simulink model "TST_RmtAPP_ChkSig"  (R2016b)
settings: Solver=FixedStepDiscrete  StartTime=0.0  StopTime=simTime  FixedStep=sampleTime  RelTol=1e-3
values from neighbouring files (symbols this model uses):
  testCase = 1    [initTST_RmtAPP_ChkSig_001.m]    (also in initTST_RmtAPP_ChkSig_002.m = 2; initTST_RmtAPP_ChkSig_003.m = 3; initTST_RmtAPP_ChkSig_004.m = 4; initTST_RmtAPP_ChkSig_005.m = 5)
libraries: simulink x11, UnitTest_Lib x5
settings Model: Creator=bianxuyin  LastModifiedBy=bianxuyin
settings DebuggingCC: SignalRangeChecking=error

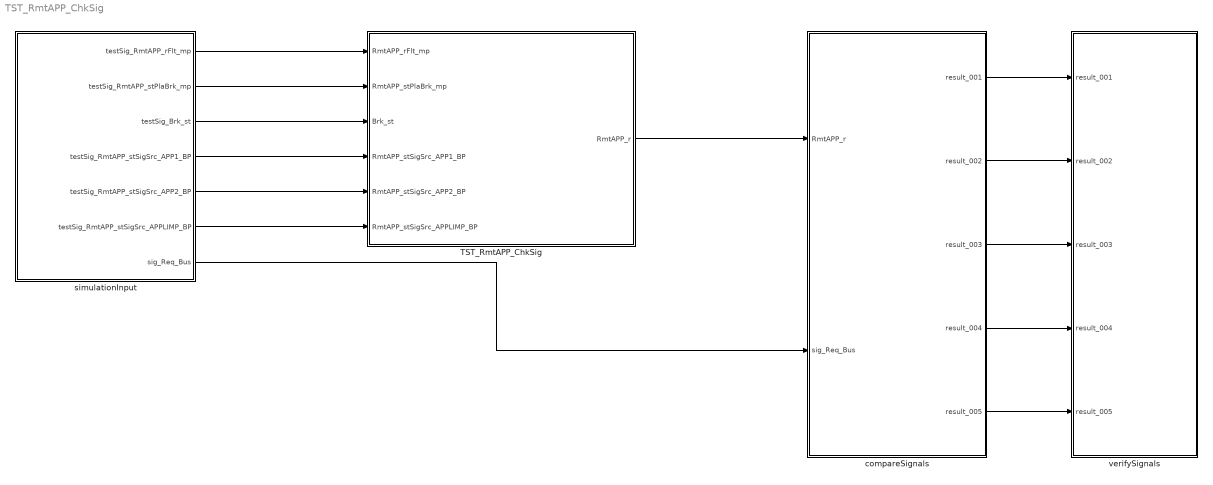
== system TST_RmtAPP_ChkSig ==
  TST_RmtAPP_ChkSig : Subsystem
  compareSignals : Subsystem
  simulationInput : Subsystem
  verifySignals : Subsystem
  wires:
  simulationInput/1(testSig_RmtAPP_rFlt_mp) -> TST_RmtAPP_ChkSig/1(RmtAPP_rFlt_mp)
  simulationInput/2(testSig_RmtAPP_stPlaBrk_mp) -> TST_RmtAPP_ChkSig/2(RmtAPP_stPlaBrk_mp)
  simulationInput/3(testSig_Brk_st) -> TST_RmtAPP_ChkSig/3(Brk_st)
  simulationInput/4(testSig_RmtAPP_stSigSrc_APP1_BP) -> TST_RmtAPP_ChkSig/4(RmtAPP_stSigSrc_APP1_BP)
  simulationInput/5(testSig_RmtAPP_stSigSrc_APP2_BP) -> TST_RmtAPP_ChkSig/5(RmtAPP_stSigSrc_APP2_BP)
  simulationInput/6(testSig_RmtAPP_stSigSrc_APPLIMP_BP) -> TST_RmtAPP_ChkSig/6(RmtAPP_stSigSrc_APPLIMP_BP)
  TST_RmtAPP_ChkSig/1(RmtAPP_r) -> compareSignals/1(RmtAPP_r)
  simulationInput/7(sig_Req_Bus) -> compareSignals/2(sig_Req_Bus)
  compareSignals/1(result_001) -> verifySignals/1(result_001)
  compareSignals/2(result_002) -> verifySignals/2(result_002)
  compareSignals/3(result_003) -> verifySignals/3(result_003)
  compareSignals/4(result_004) -> verifySignals/4(result_004)
  compareSignals/5(result_005) -> verifySignals/5(result_005)

== system TST_RmtAPP_ChkSig/TST_RmtAPP_ChkSig ==
  RmtAPP_rFlt_mp : Inport
  RmtAPP_stPlaBrk_mp : Inport  Port=2
  Brk_st : Inport  Port=3
  RmtAPP_stSigSrc_APP1_BP : Inport  Port=4
  RmtAPP_stSigSrc_APP2_BP : Inport  Port=5
  RmtAPP_stSigSrc_APPLIMP_BP : Inport  Port=6
  Function_Call : simulink/Ports & Subsystems/Function-Call Generator  sample_time=sampleTime  numberOfIterations=1
  RmtAPP_ChkSig : ModelReference  ModelNameDialog=RmtAPP_ChkSig  SimulationMode=Normal  ModelReferenceVersion=1.13  TriggerPortName=function  TriggerPortTriggerType=function-call  TriggerPortStatesWhenEnabling=held
  RmtAPP_r : Outport
  wires:
  Function_Call/1 -> RmtAPP_ChkSig/Trigger
  RmtAPP_rFlt_mp/1 -> RmtAPP_ChkSig/1
  RmtAPP_stPlaBrk_mp/1 -> RmtAPP_ChkSig/2
  Brk_st/1 -> RmtAPP_ChkSig/3
  RmtAPP_stSigSrc_APP1_BP/1 -> RmtAPP_ChkSig/4
  RmtAPP_stSigSrc_APP2_BP/1 -> RmtAPP_ChkSig/5
  RmtAPP_stSigSrc_APPLIMP_BP/1 -> RmtAPP_ChkSig/6
  RmtAPP_ChkSig/1 -> RmtAPP_r/1

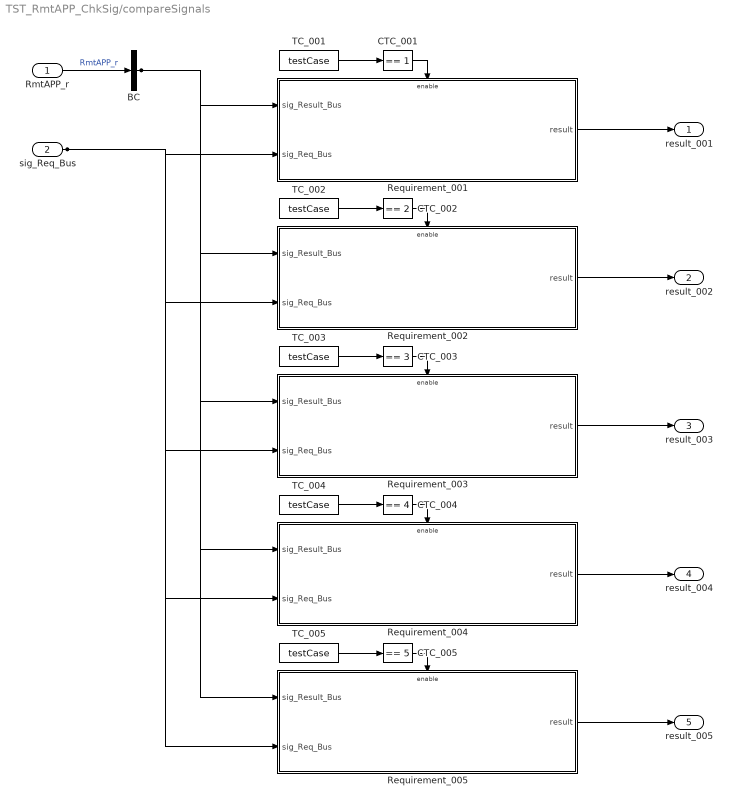
== system TST_RmtAPP_ChkSig/compareSignals ==
  RmtAPP_r : Inport
  sig_Req_Bus : Inport  Port=2
  BC : BusCreator  Inputs=1
  CTC_001 : simulink/Logic and Bit Operations/Compare To Constant  relop===  const=1  OutDataTypeStr=boolean
  CTC_002 : simulink/Logic and Bit Operations/Compare To Constant  relop===  const=2  OutDataTypeStr=boolean
  CTC_003 : simulink/Logic and Bit Operations/Compare To Constant  relop===  const=3  OutDataTypeStr=boolean
  CTC_004 : simulink/Logic and Bit Operations/Compare To Constant  relop===  const=4  OutDataTypeStr=boolean
  CTC_005 : simulink/Logic and Bit Operations/Compare To Constant  relop===  const=5  OutDataTypeStr=boolean
  Requirement_001 : Subsystem
  Requirement_002 : Subsystem
  Requirement_003 : Subsystem
  Requirement_004 : Subsystem
  Requirement_005 : Subsystem
  TC_001 : Constant  Value=testCase
  TC_002 : Constant  Value=testCase
  TC_003 : Constant  Value=testCase
  TC_004 : Constant  Value=testCase
  TC_005 : Constant  Value=testCase
  result_001 : Outport
  result_002 : Outport  Port=2
  result_003 : Outport  Port=3
  result_004 : Outport  Port=4
  result_005 : Outport  Port=5
  wires:
  RmtAPP_r/1 -> BC/1  "RmtAPP_r"
  TC_001/1 -> CTC_001/1
  CTC_001/1 -> Requirement_001/Enable
  sig_Req_Bus/1 -> Requirement_001/2(sig_Req_Bus), Requirement_002/2(sig_Req_Bus), Requirement_003/2(sig_Req_Bus), Requirement_004/2(sig_Req_Bus), Requirement_005/2(sig_Req_Bus)
  BC/1 -> Requirement_001/1(sig_Result_Bus), Requirement_002/1(sig_Result_Bus), Requirement_003/1(sig_Result_Bus), Requirement_004/1(sig_Result_Bus), Requirement_005/1(sig_Result_Bus)
  Requirement_001/1(result) -> result_001/1
  TC_002/1 -> CTC_002/1
  CTC_002/1 -> Requirement_002/Enable
  Requirement_002/1(result) -> result_002/1
  TC_003/1 -> CTC_003/1
  CTC_003/1 -> Requirement_003/Enable
  Requirement_003/1(result) -> result_003/1
  TC_004/1 -> CTC_004/1
  CTC_004/1 -> Requirement_004/Enable
  Requirement_004/1(result) -> result_004/1
  TC_005/1 -> CTC_005/1
  CTC_005/1 -> Requirement_005/Enable
  Requirement_005/1(result) -> result_005/1

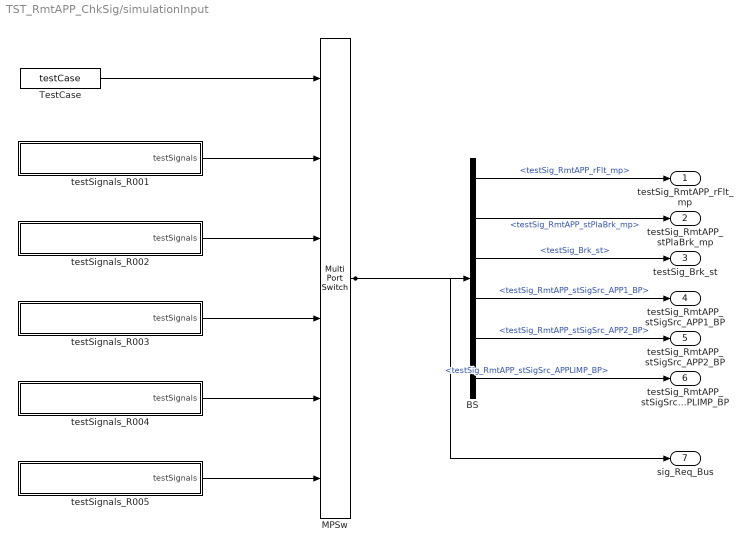
== system TST_RmtAPP_ChkSig/simulationInput ==
  BS : BusSelector  OutputSignals=testSig_RmtAPP_rFlt_mp,testSig_RmtAPP_stPlaBrk_mp,testSig_Brk_st,testSig_RmtAPP_stSigSrc_APP1_BP,testSig_RmtAPP_stSigSrc_APP2_BP,testSig_RmtAPP_stSigSrc_APPLIMP_BP
  MPSw : MultiPortSwitch  Inputs=5  SaturateOnIntegerOverflow=on  InputSameDT=on
  TestCase : Constant  Value=testCase
  testSignals_R001 : Subsystem
  testSignals_R002 : Subsystem
  testSignals_R003 : Subsystem
  testSignals_R004 : Subsystem
  testSignals_R005 : Subsystem
  testSig_RmtAPP_rFlt_mp : Outport
  testSig_RmtAPP_stPlaBrk_mp : Outport  Port=2
  testSig_Brk_st : Outport  Port=3
  testSig_RmtAPP_stSigSrc_APP1_BP : Outport  Port=4
  testSig_RmtAPP_stSigSrc_APP2_BP : Outport  Port=5
  testSig_RmtAPP_stSigSrc_APPLIMP_BP : Outport  Port=6
  sig_Req_Bus : Outport  Port=7
  wires:
  BS/1 -> testSig_RmtAPP_rFlt_mp/1  "<testSig_RmtAPP_rFlt_mp>"
  BS/2 -> testSig_RmtAPP_stPlaBrk_mp/1  "<testSig_RmtAPP_stPlaBrk_mp>"
  BS/3 -> testSig_Brk_st/1  "<testSig_Brk_st>"
  BS/4 -> testSig_RmtAPP_stSigSrc_APP1_BP/1  "<testSig_RmtAPP_stSigSrc_APP1_BP>"
  BS/5 -> testSig_RmtAPP_stSigSrc_APP2_BP/1  "<testSig_RmtAPP_stSigSrc_APP2_BP>"
  BS/6 -> testSig_RmtAPP_stSigSrc_APPLIMP_BP/1  "<testSig_RmtAPP_stSigSrc_APPLIMP_BP>"
  MPSw/1 -> BS/1, sig_Req_Bus/1
  TestCase/1 -> MPSw/1
  testSignals_R001/1(testSignals) -> MPSw/2
  testSignals_R002/1(testSignals) -> MPSw/3
  testSignals_R003/1(testSignals) -> MPSw/4
  testSignals_R004/1(testSignals) -> MPSw/5
  testSignals_R005/1(testSignals) -> MPSw/6

== system TST_RmtAPP_ChkSig/verifySignals ==
  result_001 : Inport
  result_002 : Inport  Port=2
  result_003 : Inport  Port=3
  result_004 : Inport  Port=4
  result_005 : Inport  Port=5
  Assertion_001 : Assertion  Enabled=off
  Assertion_002 : Assertion  Enabled=off
  Assertion_003 : Assertion  Enabled=off
  Assertion_004 : Assertion  Enabled=off
  Assertion_005 : Assertion  Enabled=off
  wires:
  result_001/1 -> Assertion_001/1
  result_002/1 -> Assertion_002/1
  result_003/1 -> Assertion_003/1
  result_004/1 -> Assertion_004/1
  result_005/1 -> Assertion_005/1

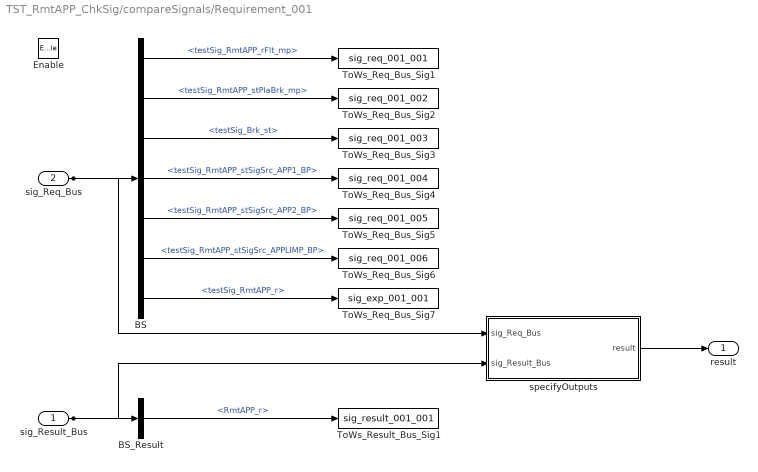
== system TST_RmtAPP_ChkSig/compareSignals/Requirement_001 ==
  sig_Result_Bus : Inport
  sig_Req_Bus : Inport  Port=2
  Enable : EnablePort
  BS : BusSelector  OutputSignals=testSig_RmtAPP_rFlt_mp,testSig_RmtAPP_stPlaBrk_mp,testSig_Brk_st,testSig_RmtAPP_stSigSrc_APP1_BP,testSig_RmtAPP_stSigSrc_APP2_BP,testSig_RmtAPP_stSigSrc_APPLIMP_BP,testSig_RmtAPP_r
  BS_Result : BusSelector  OutputSignals=RmtAPP_r
  ToWs_Req_Bus_Sig1 : ToWorkspace  VariableName=sig_req_001_001  SaveFormat=Structure With Time
  ToWs_Req_Bus_Sig2 : ToWorkspace  VariableName=sig_req_001_002  SaveFormat=Structure With Time
  ToWs_Req_Bus_Sig3 : ToWorkspace  VariableName=sig_req_001_003  SaveFormat=Structure With Time
  ToWs_Req_Bus_Sig4 : ToWorkspace  VariableName=sig_req_001_004  SaveFormat=Structure With Time
  ToWs_Req_Bus_Sig5 : ToWorkspace  VariableName=sig_req_001_005  SaveFormat=Structure With Time
  ToWs_Req_Bus_Sig6 : ToWorkspace  VariableName=sig_req_001_006  SaveFormat=Structure With Time
  ToWs_Req_Bus_Sig7 : ToWorkspace  VariableName=sig_exp_001_001  SaveFormat=Structure With Time
  ToWs_Result_Bus_Sig1 : ToWorkspace  VariableName=sig_result_001_001  SaveFormat=Structure With Time
  specifyOutputs : Subsystem
  result : Outport
  wires:
  sig_Req_Bus/1 -> BS/1, specifyOutputs/1(sig_Req_Bus)
  BS/1 -> ToWs_Req_Bus_Sig1/1  "<testSig_RmtAPP_rFlt_mp>"
  BS/2 -> ToWs_Req_Bus_Sig2/1  "<testSig_RmtAPP_stPlaBrk_mp>"
  BS/3 -> ToWs_Req_Bus_Sig3/1  "<testSig_Brk_st>"
  BS/4 -> ToWs_Req_Bus_Sig4/1  "<testSig_RmtAPP_stSigSrc_APP1_BP>"
  BS/5 -> ToWs_Req_Bus_Sig5/1  "<testSig_RmtAPP_stSigSrc_APP2_BP>"
  BS/6 -> ToWs_Req_Bus_Sig6/1  "<testSig_RmtAPP_stSigSrc_APPLIMP_BP>"
  BS/7 -> ToWs_Req_Bus_Sig7/1  "<testSig_RmtAPP_r>"
  sig_Result_Bus/1 -> BS_Result/1, specifyOutputs/2(sig_Result_Bus)
  BS_Result/1 -> ToWs_Result_Bus_Sig1/1  "<RmtAPP_r>"
  specifyOutputs/1(result) -> result/1

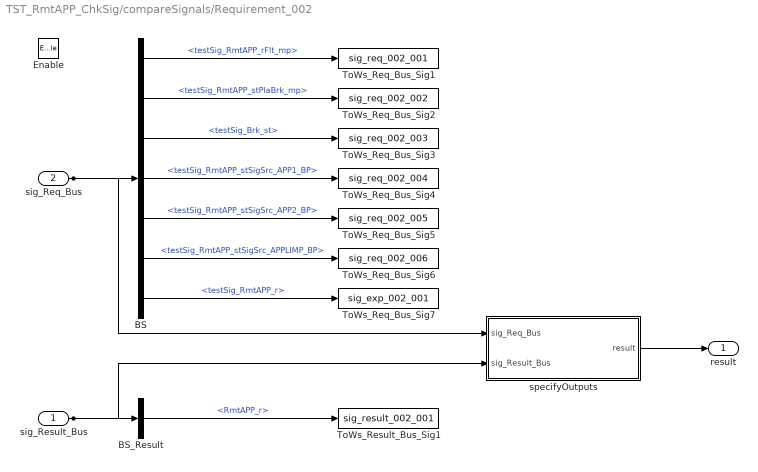
== system TST_RmtAPP_ChkSig/compareSignals/Requirement_002 ==
  sig_Result_Bus : Inport
  sig_Req_Bus : Inport  Port=2
  Enable : EnablePort
  BS : BusSelector  OutputSignals=testSig_RmtAPP_rFlt_mp,testSig_RmtAPP_stPlaBrk_mp,testSig_Brk_st,testSig_RmtAPP_stSigSrc_APP1_BP,testSig_RmtAPP_stSigSrc_APP2_BP,testSig_RmtAPP_stSigSrc_APPLIMP_BP,testSig_RmtAPP_r
  BS_Result : BusSelector  OutputSignals=RmtAPP_r
  ToWs_Req_Bus_Sig1 : ToWorkspace  VariableName=sig_req_002_001  SaveFormat=Structure With Time
  ToWs_Req_Bus_Sig2 : ToWorkspace  VariableName=sig_req_002_002  SaveFormat=Structure With Time
  ToWs_Req_Bus_Sig3 : ToWorkspace  VariableName=sig_req_002_003  SaveFormat=Structure With Time
  ToWs_Req_Bus_Sig4 : ToWorkspace  VariableName=sig_req_002_004  SaveFormat=Structure With Time
  ToWs_Req_Bus_Sig5 : ToWorkspace  VariableName=sig_req_002_005  SaveFormat=Structure With Time
  ToWs_Req_Bus_Sig6 : ToWorkspace  VariableName=sig_req_002_006  SaveFormat=Structure With Time
  ToWs_Req_Bus_Sig7 : ToWorkspace  VariableName=sig_exp_002_001  SaveFormat=Structure With Time
  ToWs_Result_Bus_Sig1 : ToWorkspace  VariableName=sig_result_002_001  SaveFormat=Structure With Time
  specifyOutputs : Subsystem
  result : Outport
  wires:
  sig_Req_Bus/1 -> BS/1, specifyOutputs/1(sig_Req_Bus)
  BS/1 -> ToWs_Req_Bus_Sig1/1  "<testSig_RmtAPP_rFlt_mp>"
  BS/2 -> ToWs_Req_Bus_Sig2/1  "<testSig_RmtAPP_stPlaBrk_mp>"
  BS/3 -> ToWs_Req_Bus_Sig3/1  "<testSig_Brk_st>"
  BS/4 -> ToWs_Req_Bus_Sig4/1  "<testSig_RmtAPP_stSigSrc_APP1_BP>"
  BS/5 -> ToWs_Req_Bus_Sig5/1  "<testSig_RmtAPP_stSigSrc_APP2_BP>"
  BS/6 -> ToWs_Req_Bus_Sig6/1  "<testSig_RmtAPP_stSigSrc_APPLIMP_BP>"
  BS/7 -> ToWs_Req_Bus_Sig7/1  "<testSig_RmtAPP_r>"
  sig_Result_Bus/1 -> BS_Result/1, specifyOutputs/2(sig_Result_Bus)
  BS_Result/1 -> ToWs_Result_Bus_Sig1/1  "<RmtAPP_r>"
  specifyOutputs/1(result) -> result/1

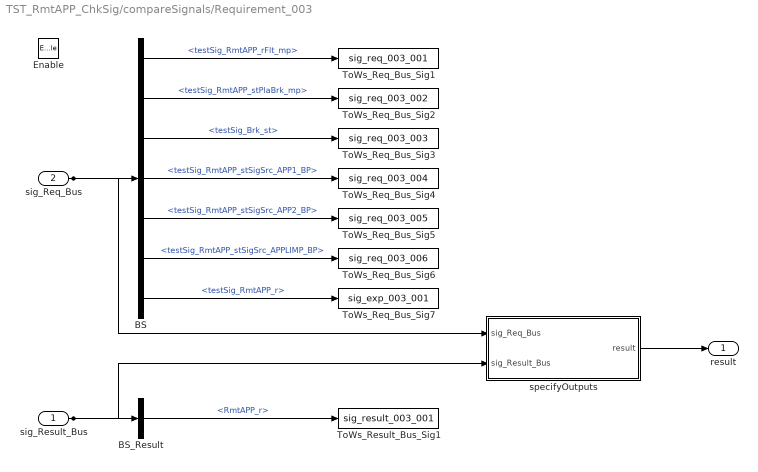
== system TST_RmtAPP_ChkSig/compareSignals/Requirement_003 ==
  sig_Result_Bus : Inport
  sig_Req_Bus : Inport  Port=2
  Enable : EnablePort
  BS : BusSelector  OutputSignals=testSig_RmtAPP_rFlt_mp,testSig_RmtAPP_stPlaBrk_mp,testSig_Brk_st,testSig_RmtAPP_stSigSrc_APP1_BP,testSig_RmtAPP_stSigSrc_APP2_BP,testSig_RmtAPP_stSigSrc_APPLIMP_BP,testSig_RmtAPP_r
  BS_Result : BusSelector  OutputSignals=RmtAPP_r
  ToWs_Req_Bus_Sig1 : ToWorkspace  VariableName=sig_req_003_001  SaveFormat=Structure With Time
  ToWs_Req_Bus_Sig2 : ToWorkspace  VariableName=sig_req_003_002  SaveFormat=Structure With Time
  ToWs_Req_Bus_Sig3 : ToWorkspace  VariableName=sig_req_003_003  SaveFormat=Structure With Time
  ToWs_Req_Bus_Sig4 : ToWorkspace  VariableName=sig_req_003_004  SaveFormat=Structure With Time
  ToWs_Req_Bus_Sig5 : ToWorkspace  VariableName=sig_req_003_005  SaveFormat=Structure With Time
  ToWs_Req_Bus_Sig6 : ToWorkspace  VariableName=sig_req_003_006  SaveFormat=Structure With Time
  ToWs_Req_Bus_Sig7 : ToWorkspace  VariableName=sig_exp_003_001  SaveFormat=Structure With Time
  ToWs_Result_Bus_Sig1 : ToWorkspace  VariableName=sig_result_003_001  SaveFormat=Structure With Time
  specifyOutputs : Subsystem
  result : Outport
  wires:
  sig_Req_Bus/1 -> BS/1, specifyOutputs/1(sig_Req_Bus)
  BS/1 -> ToWs_Req_Bus_Sig1/1  "<testSig_RmtAPP_rFlt_mp>"
  BS/2 -> ToWs_Req_Bus_Sig2/1  "<testSig_RmtAPP_stPlaBrk_mp>"
  BS/3 -> ToWs_Req_Bus_Sig3/1  "<testSig_Brk_st>"
  BS/4 -> ToWs_Req_Bus_Sig4/1  "<testSig_RmtAPP_stSigSrc_APP1_BP>"
  BS/5 -> ToWs_Req_Bus_Sig5/1  "<testSig_RmtAPP_stSigSrc_APP2_BP>"
  BS/6 -> ToWs_Req_Bus_Sig6/1  "<testSig_RmtAPP_stSigSrc_APPLIMP_BP>"
  BS/7 -> ToWs_Req_Bus_Sig7/1  "<testSig_RmtAPP_r>"
  sig_Result_Bus/1 -> BS_Result/1, specifyOutputs/2(sig_Result_Bus)
  BS_Result/1 -> ToWs_Result_Bus_Sig1/1  "<RmtAPP_r>"
  specifyOutputs/1(result) -> result/1

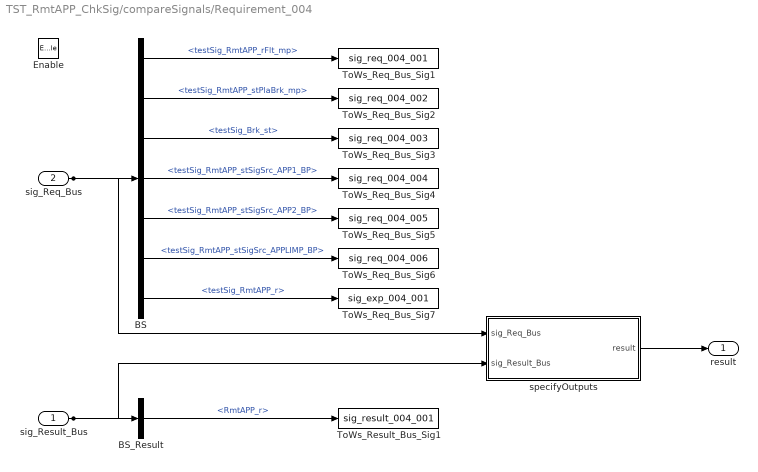
== system TST_RmtAPP_ChkSig/compareSignals/Requirement_004 ==
  sig_Result_Bus : Inport
  sig_Req_Bus : Inport  Port=2
  Enable : EnablePort
  BS : BusSelector  OutputSignals=testSig_RmtAPP_rFlt_mp,testSig_RmtAPP_stPlaBrk_mp,testSig_Brk_st,testSig_RmtAPP_stSigSrc_APP1_BP,testSig_RmtAPP_stSigSrc_APP2_BP,testSig_RmtAPP_stSigSrc_APPLIMP_BP,testSig_RmtAPP_r
  BS_Result : BusSelector  OutputSignals=RmtAPP_r
  ToWs_Req_Bus_Sig1 : ToWorkspace  VariableName=sig_req_004_001  SaveFormat=Structure With Time
  ToWs_Req_Bus_Sig2 : ToWorkspace  VariableName=sig_req_004_002  SaveFormat=Structure With Time
  ToWs_Req_Bus_Sig3 : ToWorkspace  VariableName=sig_req_004_003  SaveFormat=Structure With Time
  ToWs_Req_Bus_Sig4 : ToWorkspace  VariableName=sig_req_004_004  SaveFormat=Structure With Time
  ToWs_Req_Bus_Sig5 : ToWorkspace  VariableName=sig_req_004_005  SaveFormat=Structure With Time
  ToWs_Req_Bus_Sig6 : ToWorkspace  VariableName=sig_req_004_006  SaveFormat=Structure With Time
  ToWs_Req_Bus_Sig7 : ToWorkspace  VariableName=sig_exp_004_001  SaveFormat=Structure With Time
  ToWs_Result_Bus_Sig1 : ToWorkspace  VariableName=sig_result_004_001  SaveFormat=Structure With Time
  specifyOutputs : Subsystem
  result : Outport
  wires:
  sig_Req_Bus/1 -> BS/1, specifyOutputs/1(sig_Req_Bus)
  BS/1 -> ToWs_Req_Bus_Sig1/1  "<testSig_RmtAPP_rFlt_mp>"
  BS/2 -> ToWs_Req_Bus_Sig2/1  "<testSig_RmtAPP_stPlaBrk_mp>"
  BS/3 -> ToWs_Req_Bus_Sig3/1  "<testSig_Brk_st>"
  BS/4 -> ToWs_Req_Bus_Sig4/1  "<testSig_RmtAPP_stSigSrc_APP1_BP>"
  BS/5 -> ToWs_Req_Bus_Sig5/1  "<testSig_RmtAPP_stSigSrc_APP2_BP>"
  BS/6 -> ToWs_Req_Bus_Sig6/1  "<testSig_RmtAPP_stSigSrc_APPLIMP_BP>"
  BS/7 -> ToWs_Req_Bus_Sig7/1  "<testSig_RmtAPP_r>"
  sig_Result_Bus/1 -> BS_Result/1, specifyOutputs/2(sig_Result_Bus)
  BS_Result/1 -> ToWs_Result_Bus_Sig1/1  "<RmtAPP_r>"
  specifyOutputs/1(result) -> result/1

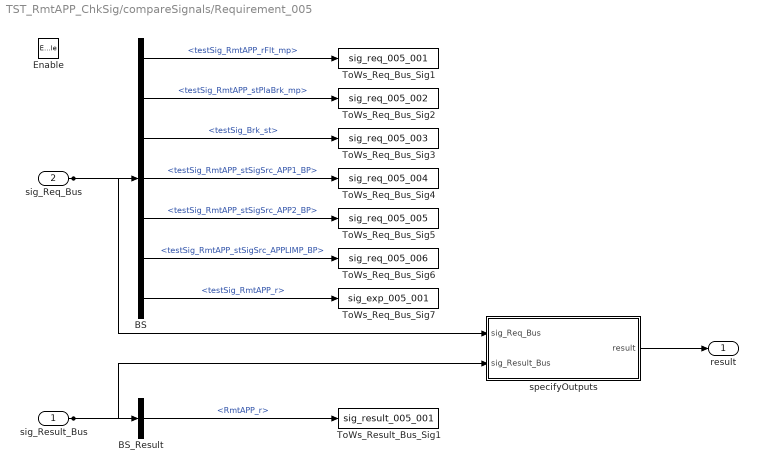
== system TST_RmtAPP_ChkSig/compareSignals/Requirement_005 ==
  sig_Result_Bus : Inport
  sig_Req_Bus : Inport  Port=2
  Enable : EnablePort
  BS : BusSelector  OutputSignals=testSig_RmtAPP_rFlt_mp,testSig_RmtAPP_stPlaBrk_mp,testSig_Brk_st,testSig_RmtAPP_stSigSrc_APP1_BP,testSig_RmtAPP_stSigSrc_APP2_BP,testSig_RmtAPP_stSigSrc_APPLIMP_BP,testSig_RmtAPP_r
  BS_Result : BusSelector  OutputSignals=RmtAPP_r
  ToWs_Req_Bus_Sig1 : ToWorkspace  VariableName=sig_req_005_001  SaveFormat=Structure With Time
  ToWs_Req_Bus_Sig2 : ToWorkspace  VariableName=sig_req_005_002  SaveFormat=Structure With Time
  ToWs_Req_Bus_Sig3 : ToWorkspace  VariableName=sig_req_005_003  SaveFormat=Structure With Time
  ToWs_Req_Bus_Sig4 : ToWorkspace  VariableName=sig_req_005_004  SaveFormat=Structure With Time
  ToWs_Req_Bus_Sig5 : ToWorkspace  VariableName=sig_req_005_005  SaveFormat=Structure With Time
  ToWs_Req_Bus_Sig6 : ToWorkspace  VariableName=sig_req_005_006  SaveFormat=Structure With Time
  ToWs_Req_Bus_Sig7 : ToWorkspace  VariableName=sig_exp_005_001  SaveFormat=Structure With Time
  ToWs_Result_Bus_Sig1 : ToWorkspace  VariableName=sig_result_005_001  SaveFormat=Structure With Time
  specifyOutputs : Subsystem
  result : Outport
  wires:
  sig_Req_Bus/1 -> BS/1, specifyOutputs/1(sig_Req_Bus)
  BS/1 -> ToWs_Req_Bus_Sig1/1  "<testSig_RmtAPP_rFlt_mp>"
  BS/2 -> ToWs_Req_Bus_Sig2/1  "<testSig_RmtAPP_stPlaBrk_mp>"
  BS/3 -> ToWs_Req_Bus_Sig3/1  "<testSig_Brk_st>"
  BS/4 -> ToWs_Req_Bus_Sig4/1  "<testSig_RmtAPP_stSigSrc_APP1_BP>"
  BS/5 -> ToWs_Req_Bus_Sig5/1  "<testSig_RmtAPP_stSigSrc_APP2_BP>"
  BS/6 -> ToWs_Req_Bus_Sig6/1  "<testSig_RmtAPP_stSigSrc_APPLIMP_BP>"
  BS/7 -> ToWs_Req_Bus_Sig7/1  "<testSig_RmtAPP_r>"
  sig_Result_Bus/1 -> BS_Result/1, specifyOutputs/2(sig_Result_Bus)
  BS_Result/1 -> ToWs_Result_Bus_Sig1/1  "<RmtAPP_r>"
  specifyOutputs/1(result) -> result/1

== system TST_RmtAPP_ChkSig/simulationInput/testSignals_R001 ==
  BC : BusCreator  Inputs=7
  spec_Brk_st : FromWorkspace  VariableName=testSig_Brk_st  Interpolate=off  OutputAfterFinalValue=Holding final value
  spec_RmtAPP_r : FromWorkspace  VariableName=testSig_RmtAPP_r  Interpolate=off  OutputAfterFinalValue=Holding final value
  spec_RmtAPP_rFlt_mp : FromWorkspace  VariableName=testSig_RmtAPP_rFlt_mp  Interpolate=off  OutputAfterFinalValue=Holding final value
  spec_RmtAPP_stPlaBrk_mp : FromWorkspace  VariableName=testSig_RmtAPP_stPlaBrk_mp  Interpolate=off  OutputAfterFinalValue=Holding final value
  spec_RmtAPP_stSigSrc_APP1_BP : FromWorkspace  VariableName=testSig_RmtAPP_stSigSrc_APP1_BP  Interpolate=off  OutputAfterFinalValue=Holding final value
  spec_RmtAPP_stSigSrc_APP2_BP : FromWorkspace  VariableName=testSig_RmtAPP_stSigSrc_APP2_BP  Interpolate=off  OutputAfterFinalValue=Holding final value
  spec_RmtAPP_stSigSrc_APPLIMP_BP : FromWorkspace  VariableName=testSig_RmtAPP_stSigSrc_APPLIMP_BP  Interpolate=off  OutputAfterFinalValue=Holding final value
  testSignals : Outport
  wires:
  BC/1 -> testSignals/1
  spec_RmtAPP_rFlt_mp/1 -> BC/1  "testSig_RmtAPP_rFlt_mp"
  spec_RmtAPP_stPlaBrk_mp/1 -> BC/2  "testSig_RmtAPP_stPlaBrk_mp"
  spec_Brk_st/1 -> BC/3  "testSig_Brk_st"
  spec_RmtAPP_stSigSrc_APP1_BP/1 -> BC/4  "testSig_RmtAPP_stSigSrc_APP1_BP"
  spec_RmtAPP_stSigSrc_APP2_BP/1 -> BC/5  "testSig_RmtAPP_stSigSrc_APP2_BP"
  spec_RmtAPP_stSigSrc_APPLIMP_BP/1 -> BC/6  "testSig_RmtAPP_stSigSrc_APPLIMP_BP"
  spec_RmtAPP_r/1 -> BC/7  "testSig_RmtAPP_r"

== system TST_RmtAPP_ChkSig/simulationInput/testSignals_R002 ==
  BC : BusCreator  Inputs=7
  spec_Brk_st : FromWorkspace  VariableName=testSig_Brk_st  Interpolate=off  OutputAfterFinalValue=Holding final value
  spec_RmtAPP_r : FromWorkspace  VariableName=testSig_RmtAPP_r  Interpolate=off  OutputAfterFinalValue=Holding final value
  spec_RmtAPP_rFlt_mp : FromWorkspace  VariableName=testSig_RmtAPP_rFlt_mp  Interpolate=off  OutputAfterFinalValue=Holding final value
  spec_RmtAPP_stPlaBrk_mp : FromWorkspace  VariableName=testSig_RmtAPP_stPlaBrk_mp  Interpolate=off  OutputAfterFinalValue=Holding final value
  spec_RmtAPP_stSigSrc_APP1_BP : FromWorkspace  VariableName=testSig_RmtAPP_stSigSrc_APP1_BP  Interpolate=off  OutputAfterFinalValue=Holding final value
  spec_RmtAPP_stSigSrc_APP2_BP : FromWorkspace  VariableName=testSig_RmtAPP_stSigSrc_APP2_BP  Interpolate=off  OutputAfterFinalValue=Holding final value
  spec_RmtAPP_stSigSrc_APPLIMP_BP : FromWorkspace  VariableName=testSig_RmtAPP_stSigSrc_APPLIMP_BP  Interpolate=off  OutputAfterFinalValue=Holding final value
  testSignals : Outport
  wires:
  BC/1 -> testSignals/1
  spec_RmtAPP_rFlt_mp/1 -> BC/1  "testSig_RmtAPP_rFlt_mp"
  spec_RmtAPP_stPlaBrk_mp/1 -> BC/2  "testSig_RmtAPP_stPlaBrk_mp"
  spec_Brk_st/1 -> BC/3  "testSig_Brk_st"
  spec_RmtAPP_stSigSrc_APP1_BP/1 -> BC/4  "testSig_RmtAPP_stSigSrc_APP1_BP"
  spec_RmtAPP_stSigSrc_APP2_BP/1 -> BC/5  "testSig_RmtAPP_stSigSrc_APP2_BP"
  spec_RmtAPP_stSigSrc_APPLIMP_BP/1 -> BC/6  "testSig_RmtAPP_stSigSrc_APPLIMP_BP"
  spec_RmtAPP_r/1 -> BC/7  "testSig_RmtAPP_r"

== system TST_RmtAPP_ChkSig/simulationInput/testSignals_R003 ==
  BC : BusCreator  Inputs=7
  spec_Brk_st : FromWorkspace  VariableName=testSig_Brk_st  Interpolate=off  OutputAfterFinalValue=Holding final value
  spec_RmtAPP_r : FromWorkspace  VariableName=testSig_RmtAPP_r  Interpolate=off  OutputAfterFinalValue=Holding final value
  spec_RmtAPP_rFlt_mp : FromWorkspace  VariableName=testSig_RmtAPP_rFlt_mp  Interpolate=off  OutputAfterFinalValue=Holding final value
  spec_RmtAPP_stPlaBrk_mp : FromWorkspace  VariableName=testSig_RmtAPP_stPlaBrk_mp  Interpolate=off  OutputAfterFinalValue=Holding final value
  spec_RmtAPP_stSigSrc_APP1_BP : FromWorkspace  VariableName=testSig_RmtAPP_stSigSrc_APP1_BP  Interpolate=off  OutputAfterFinalValue=Holding final value
  spec_RmtAPP_stSigSrc_APP2_BP : FromWorkspace  VariableName=testSig_RmtAPP_stSigSrc_APP2_BP  Interpolate=off  OutputAfterFinalValue=Holding final value
  spec_RmtAPP_stSigSrc_APPLIMP_BP : FromWorkspace  VariableName=testSig_RmtAPP_stSigSrc_APPLIMP_BP  Interpolate=off  OutputAfterFinalValue=Holding final value
  testSignals : Outport
  wires:
  BC/1 -> testSignals/1
  spec_RmtAPP_rFlt_mp/1 -> BC/1  "testSig_RmtAPP_rFlt_mp"
  spec_RmtAPP_stPlaBrk_mp/1 -> BC/2  "testSig_RmtAPP_stPlaBrk_mp"
  spec_Brk_st/1 -> BC/3  "testSig_Brk_st"
  spec_RmtAPP_stSigSrc_APP1_BP/1 -> BC/4  "testSig_RmtAPP_stSigSrc_APP1_BP"
  spec_RmtAPP_stSigSrc_APP2_BP/1 -> BC/5  "testSig_RmtAPP_stSigSrc_APP2_BP"
  spec_RmtAPP_stSigSrc_APPLIMP_BP/1 -> BC/6  "testSig_RmtAPP_stSigSrc_APPLIMP_BP"
  spec_RmtAPP_r/1 -> BC/7  "testSig_RmtAPP_r"

== system TST_RmtAPP_ChkSig/simulationInput/testSignals_R004 ==
  BC : BusCreator  Inputs=7
  spec_Brk_st : FromWorkspace  VariableName=testSig_Brk_st  Interpolate=off  OutputAfterFinalValue=Holding final value
  spec_RmtAPP_r : FromWorkspace  VariableName=testSig_RmtAPP_r  Interpolate=off  OutputAfterFinalValue=Holding final value
  spec_RmtAPP_rFlt_mp : FromWorkspace  VariableName=testSig_RmtAPP_rFlt_mp  Interpolate=off  OutputAfterFinalValue=Holding final value
  spec_RmtAPP_stPlaBrk_mp : FromWorkspace  VariableName=testSig_RmtAPP_stPlaBrk_mp  Interpolate=off  OutputAfterFinalValue=Holding final value
  spec_RmtAPP_stSigSrc_APP1_BP : FromWorkspace  VariableName=testSig_RmtAPP_stSigSrc_APP1_BP  Interpolate=off  OutputAfterFinalValue=Holding final value
  spec_RmtAPP_stSigSrc_APP2_BP : FromWorkspace  VariableName=testSig_RmtAPP_stSigSrc_APP2_BP  Interpolate=off  OutputAfterFinalValue=Holding final value
  spec_RmtAPP_stSigSrc_APPLIMP_BP : FromWorkspace  VariableName=testSig_RmtAPP_stSigSrc_APPLIMP_BP  Interpolate=off  OutputAfterFinalValue=Holding final value
  testSignals : Outport
  wires:
  BC/1 -> testSignals/1
  spec_RmtAPP_rFlt_mp/1 -> BC/1  "testSig_RmtAPP_rFlt_mp"
  spec_RmtAPP_stPlaBrk_mp/1 -> BC/2  "testSig_RmtAPP_stPlaBrk_mp"
  spec_Brk_st/1 -> BC/3  "testSig_Brk_st"
  spec_RmtAPP_stSigSrc_APP1_BP/1 -> BC/4  "testSig_RmtAPP_stSigSrc_APP1_BP"
  spec_RmtAPP_stSigSrc_APP2_BP/1 -> BC/5  "testSig_RmtAPP_stSigSrc_APP2_BP"
  spec_RmtAPP_stSigSrc_APPLIMP_BP/1 -> BC/6  "testSig_RmtAPP_stSigSrc_APPLIMP_BP"
  spec_RmtAPP_r/1 -> BC/7  "testSig_RmtAPP_r"

== system TST_RmtAPP_ChkSig/simulationInput/testSignals_R005 ==
  BC : BusCreator  Inputs=7
  spec_Brk_st : FromWorkspace  VariableName=testSig_Brk_st  Interpolate=off  OutputAfterFinalValue=Holding final value
  spec_RmtAPP_r : FromWorkspace  VariableName=testSig_RmtAPP_r  Interpolate=off  OutputAfterFinalValue=Holding final value
  spec_RmtAPP_rFlt_mp : FromWorkspace  VariableName=testSig_RmtAPP_rFlt_mp  Interpolate=off  OutputAfterFinalValue=Holding final value
  spec_RmtAPP_stPlaBrk_mp : FromWorkspace  VariableName=testSig_RmtAPP_stPlaBrk_mp  Interpolate=off  OutputAfterFinalValue=Holding final value
  spec_RmtAPP_stSigSrc_APP1_BP : FromWorkspace  VariableName=testSig_RmtAPP_stSigSrc_APP1_BP  Interpolate=off  OutputAfterFinalValue=Holding final value
  spec_RmtAPP_stSigSrc_APP2_BP : FromWorkspace  VariableName=testSig_RmtAPP_stSigSrc_APP2_BP  Interpolate=off  OutputAfterFinalValue=Holding final value
  spec_RmtAPP_stSigSrc_APPLIMP_BP : FromWorkspace  VariableName=testSig_RmtAPP_stSigSrc_APPLIMP_BP  Interpolate=off  OutputAfterFinalValue=Holding final value
  testSignals : Outport
  wires:
  BC/1 -> testSignals/1
  spec_RmtAPP_rFlt_mp/1 -> BC/1  "testSig_RmtAPP_rFlt_mp"
  spec_RmtAPP_stPlaBrk_mp/1 -> BC/2  "testSig_RmtAPP_stPlaBrk_mp"
  spec_Brk_st/1 -> BC/3  "testSig_Brk_st"
  spec_RmtAPP_stSigSrc_APP1_BP/1 -> BC/4  "testSig_RmtAPP_stSigSrc_APP1_BP"
  spec_RmtAPP_stSigSrc_APP2_BP/1 -> BC/5  "testSig_RmtAPP_stSigSrc_APP2_BP"
  spec_RmtAPP_stSigSrc_APPLIMP_BP/1 -> BC/6  "testSig_RmtAPP_stSigSrc_APPLIMP_BP"
  spec_RmtAPP_r/1 -> BC/7  "testSig_RmtAPP_r"

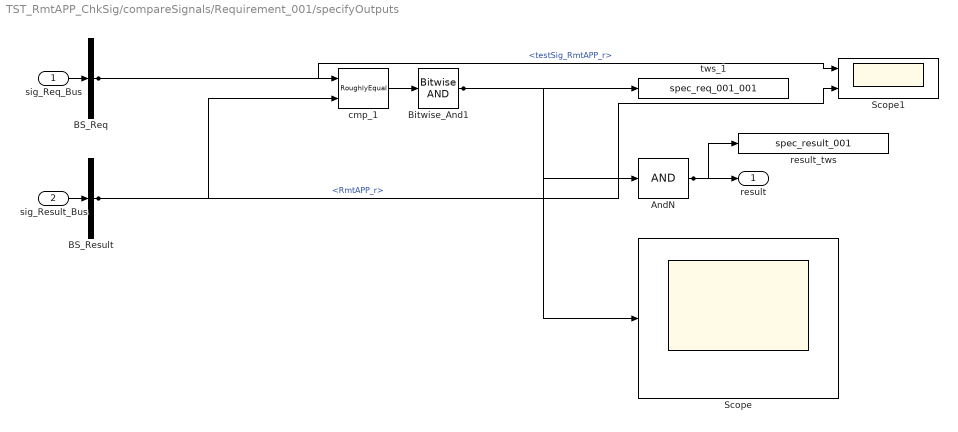
== system TST_RmtAPP_ChkSig/compareSignals/Requirement_001/specifyOutputs ==
  sig_Req_Bus : Inport
  sig_Result_Bus : Inport  Port=2
  AndN : Logic  Inputs=1
  BS_Req : BusSelector  OutputSignals=testSig_RmtAPP_r
  BS_Result : BusSelector  OutputSignals=RmtAPP_r
  Bitwise_And1 : simulink/Logic and Bit Operations/Bitwise Operator  logicop=AND  UseBitMask=off  BitMask=bin2dec('11011001')  BitMaskRealWorld=Stored Integer
  Scope : Scope
  Scope1 : Scope  NumInputPorts=2
  cmp_1 : UnitTest_Lib/RoughlyEqual  slope=0.1
  result_tws : ToWorkspace  VariableName=spec_result_001
  tws_1 : ToWorkspace  VariableName=spec_req_001_001
  result : Outport
  wires:
  sig_Req_Bus/1 -> BS_Req/1
  sig_Result_Bus/1 -> BS_Result/1
  AndN/1 -> result/1, result_tws/1
  BS_Req/1 -> cmp_1/1, Scope1/1  "<testSig_RmtAPP_r>"
  BS_Result/1 -> cmp_1/2, Scope1/2  "<RmtAPP_r>"
  cmp_1/1 -> Bitwise_And1/1
  Bitwise_And1/1 -> tws_1/1, AndN/1, Scope/1

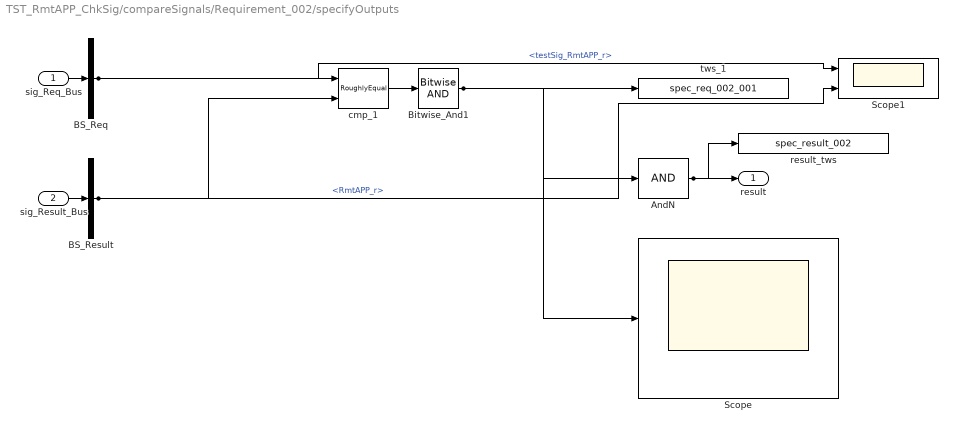
== system TST_RmtAPP_ChkSig/compareSignals/Requirement_002/specifyOutputs ==
  sig_Req_Bus : Inport
  sig_Result_Bus : Inport  Port=2
  AndN : Logic  Inputs=1
  BS_Req : BusSelector  OutputSignals=testSig_RmtAPP_r
  BS_Result : BusSelector  OutputSignals=RmtAPP_r
  Bitwise_And1 : simulink/Logic and Bit Operations/Bitwise Operator  logicop=AND  UseBitMask=off  BitMask=bin2dec('11011001')  BitMaskRealWorld=Stored Integer
  Scope : Scope
  Scope1 : Scope  NumInputPorts=2
  cmp_1 : UnitTest_Lib/RoughlyEqual  slope=0.1
  result_tws : ToWorkspace  VariableName=spec_result_002
  tws_1 : ToWorkspace  VariableName=spec_req_002_001
  result : Outport
  wires:
  sig_Req_Bus/1 -> BS_Req/1
  sig_Result_Bus/1 -> BS_Result/1
  AndN/1 -> result/1, result_tws/1
  BS_Req/1 -> cmp_1/1, Scope1/1  "<testSig_RmtAPP_r>"
  BS_Result/1 -> cmp_1/2, Scope1/2  "<RmtAPP_r>"
  cmp_1/1 -> Bitwise_And1/1
  Bitwise_And1/1 -> tws_1/1, AndN/1, Scope/1

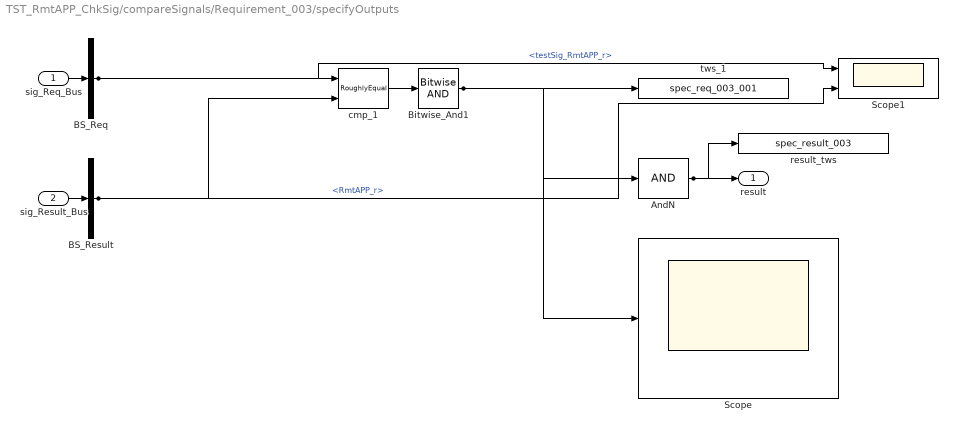
== system TST_RmtAPP_ChkSig/compareSignals/Requirement_003/specifyOutputs ==
  sig_Req_Bus : Inport
  sig_Result_Bus : Inport  Port=2
  AndN : Logic  Inputs=1
  BS_Req : BusSelector  OutputSignals=testSig_RmtAPP_r
  BS_Result : BusSelector  OutputSignals=RmtAPP_r
  Bitwise_And1 : simulink/Logic and Bit Operations/Bitwise Operator  logicop=AND  UseBitMask=off  BitMask=bin2dec('11011001')  BitMaskRealWorld=Stored Integer
  Scope : Scope
  Scope1 : Scope  NumInputPorts=2
  cmp_1 : UnitTest_Lib/RoughlyEqual  slope=0.1
  result_tws : ToWorkspace  VariableName=spec_result_003
  tws_1 : ToWorkspace  VariableName=spec_req_003_001
  result : Outport
  wires:
  sig_Req_Bus/1 -> BS_Req/1
  sig_Result_Bus/1 -> BS_Result/1
  AndN/1 -> result/1, result_tws/1
  BS_Req/1 -> cmp_1/1, Scope1/1  "<testSig_RmtAPP_r>"
  BS_Result/1 -> cmp_1/2, Scope1/2  "<RmtAPP_r>"
  cmp_1/1 -> Bitwise_And1/1
  Bitwise_And1/1 -> tws_1/1, AndN/1, Scope/1

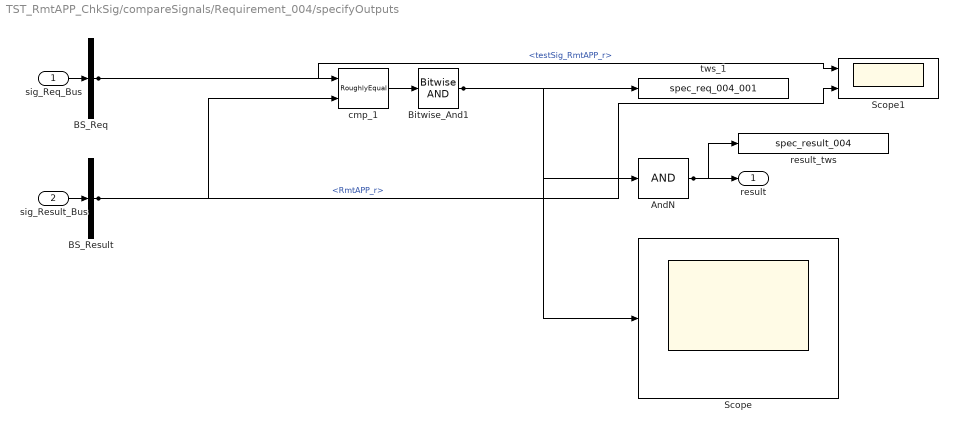
== system TST_RmtAPP_ChkSig/compareSignals/Requirement_004/specifyOutputs ==
  sig_Req_Bus : Inport
  sig_Result_Bus : Inport  Port=2
  AndN : Logic  Inputs=1
  BS_Req : BusSelector  OutputSignals=testSig_RmtAPP_r
  BS_Result : BusSelector  OutputSignals=RmtAPP_r
  Bitwise_And1 : simulink/Logic and Bit Operations/Bitwise Operator  logicop=AND  UseBitMask=off  BitMask=bin2dec('11011001')  BitMaskRealWorld=Stored Integer
  Scope : Scope
  Scope1 : Scope  NumInputPorts=2
  cmp_1 : UnitTest_Lib/RoughlyEqual  slope=0.1
  result_tws : ToWorkspace  VariableName=spec_result_004
  tws_1 : ToWorkspace  VariableName=spec_req_004_001
  result : Outport
  wires:
  sig_Req_Bus/1 -> BS_Req/1
  sig_Result_Bus/1 -> BS_Result/1
  AndN/1 -> result/1, result_tws/1
  BS_Req/1 -> cmp_1/1, Scope1/1  "<testSig_RmtAPP_r>"
  BS_Result/1 -> cmp_1/2, Scope1/2  "<RmtAPP_r>"
  cmp_1/1 -> Bitwise_And1/1
  Bitwise_And1/1 -> tws_1/1, AndN/1, Scope/1

== system TST_RmtAPP_ChkSig/compareSignals/Requirement_005/specifyOutputs ==
  sig_Req_Bus : Inport
  sig_Result_Bus : Inport  Port=2
  AndN : Logic  Inputs=1
  BS_Req : BusSelector  OutputSignals=testSig_RmtAPP_r
  BS_Result : BusSelector  OutputSignals=RmtAPP_r
  Bitwise_And1 : simulink/Logic and Bit Operations/Bitwise Operator  logicop=AND  UseBitMask=off  BitMask=bin2dec('11011001')  BitMaskRealWorld=Stored Integer
  Scope : Scope
  Scope1 : Scope  NumInputPorts=2
  cmp_1 : UnitTest_Lib/RoughlyEqual  slope=0.1
  result_tws : ToWorkspace  VariableName=spec_result_005
  tws_1 : ToWorkspace  VariableName=spec_req_005_001
  result : Outport
  wires:
  sig_Req_Bus/1 -> BS_Req/1
  sig_Result_Bus/1 -> BS_Result/1
  AndN/1 -> result/1, result_tws/1
  BS_Req/1 -> cmp_1/1, Scope1/1  "<testSig_RmtAPP_r>"
  BS_Result/1 -> cmp_1/2, Scope1/2  "<RmtAPP_r>"
  cmp_1/1 -> Bitwise_And1/1
  Bitwise_And1/1 -> tws_1/1, AndN/1, Scope/1
